simulink model "Project5_model"  (R2014b)
settings: Solver=ode5  StartTime=0.0  StopTime=2  FixedStep=0.01  RelTol=1e-3
undefined symbols (not defined in the file or in its folder): Kd, Ki, Kp
settings Model: Creator=axk7578  LastModifiedBy=axk7578

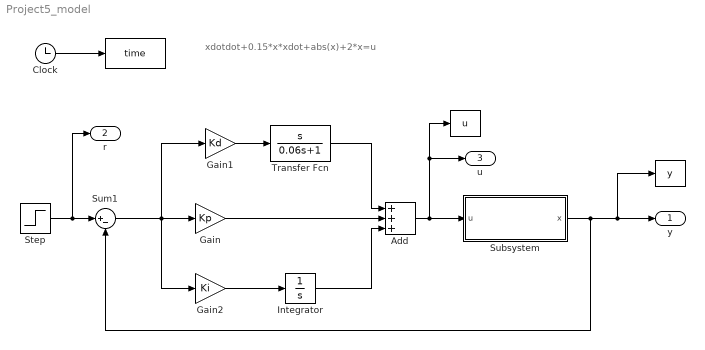
== system Project5_model ==
  note: xdotdot+0.15*x*xdot+abs(x)+2*x=u
  " " : ToWorkspace  VariableName=time  SampleTime=-1
  " " : ToWorkspace  VariableName=y  SampleTime=-1
  " " : ToWorkspace  VariableName=u  SampleTime=-1
  Add : Sum  Inputs=+++
  Clock : Clock
  Gain : Gain  Gain=Kp
  Gain1 : Gain  Gain=Kd
  Gain2 : Gain  Gain=Ki
  Integrator : Integrator
  Step : Step  Time=0  SampleTime=0
  Subsystem : Subsystem
  Sum1 : Sum  Inputs=|+-
  Transfer Fcn : TransferFcn  Numerator=[1 0]  Denominator=[0.06 1]
  y : Outport
  r : Outport  Port=2
  u : Outport  Port=3
  wires:
  Clock/1 -> " "/1
  Step/1 -> r/1, Sum1/1
  Sum1/1 -> Gain2/1, Gain1/1, Gain/1
  Gain1/1 -> Transfer Fcn/1
  Gain/1 -> Add/2
  Transfer Fcn/1 -> Add/1
  Gain2/1 -> Integrator/1
  Integrator/1 -> Add/3
  Add/1 -> u/1, " "/1, Subsystem/1(u)
  Subsystem/1(x) -> Sum1/2, " "/1, y/1

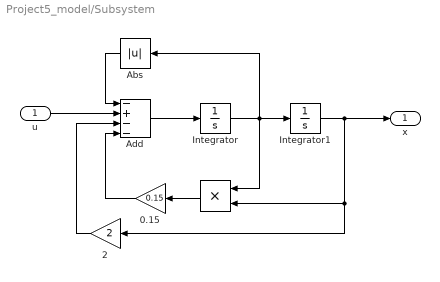
== system Project5_model/Subsystem ==
  u : Inport
  " " : Product
  0.15 : Gain  Gain=0.15
  2 : Gain  Gain=2
  Abs : Abs
  Add : Sum  Inputs=-+--
  Integrator : Integrator
  Integrator1 : Integrator
  x : Outport
  wires:
  Integrator/1 -> Abs/1, " "/1, Integrator1/1
  Integrator1/1 -> 2/1, " "/2, x/1
  Add/1 -> Integrator/1
  " "/1 -> 0.15/1
  0.15/1 -> Add/4
  u/1 -> Add/2
  Abs/1 -> Add/1
  2/1 -> Add/3
